simulink model "problem3"  (R2020b)
settings: Solver=VariableStepAuto  StartTime=0.0  StopTime=10.0  RelTol=1e-3
model workspace: external: MAT-File gain_val.mat (data not in the file)
values from neighbouring files (symbols this model uses):
  a = 0.1584    [gain_val.mat]
settings Model: ParameterArgumentNames=a  OrderedModelArguments=off  Creator=admin  LastModifiedBy=admin

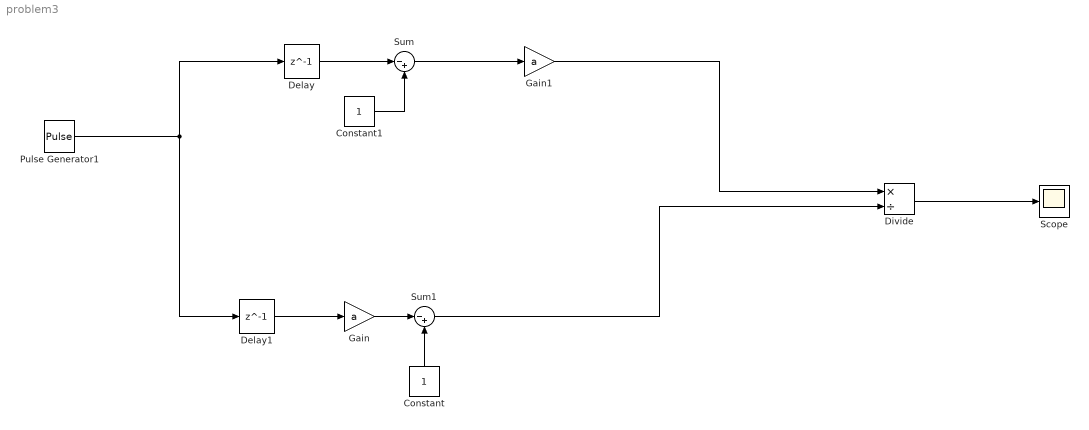
== system problem3 ==
  Constant : Constant
  Constant1 : Constant
  Delay : Delay  DelayLength=1  InitialCondition=0
  Delay1 : Delay  DelayLength=1  InitialCondition=0
  Divide : Product  Inputs=*/
  Gain : Gain  Gain=a
  Gain1 : Gain  Gain=a
  Pulse Generator1 : DiscretePulseGenerator  PulseType=Time based  Period=10  PulseWidth=5
  Scope : Scope
  Sum : Sum  Inputs=|-+
  Sum1 : Sum  Inputs=|-+
  wires:
  Pulse Generator1/1 -> Delay/1, Delay1/1
  Delay1/1 -> Gain/1
  Divide/1 -> Scope/1
  Gain1/1 -> Divide/1
  Constant/1 -> Sum1/2
  Gain/1 -> Sum1/1
  Constant1/1 -> Sum/2
  Delay/1 -> Sum/1
  Sum/1 -> Gain1/1
  Sum1/1 -> Divide/2
